simulink model "s23"  (R2019b)
settings: Solver=VariableStepAuto  StartTime=0.0  StopTime=10.0  RelTol=1e-3
values from neighbouring files (symbols this model uses):
  D = DVect(2)    [aula3.m]    (also in aula3_mica.m = Dvector(n); s23.m = 0.1)
  J = Jl + Jm    [s23.m]
  Km = 1 ,Kg = 0.1    [s23.m]
  L = 1e-3    (= 0.001)    [ex1.m]
  R = 10    [ex1.m]
undefined symbols (not defined in the file or in its folder): Kg
settings Model: Creator=Emanuel Pereira  LastModifiedBy=Emanuel Pereira

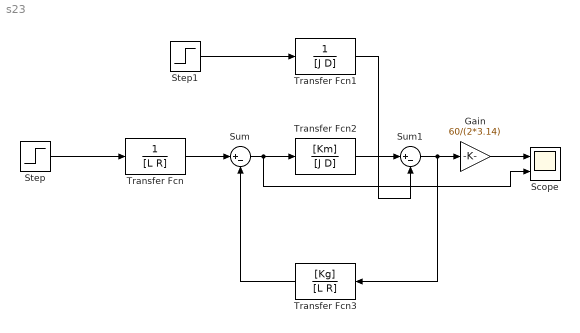
== system s23 ==
  Gain : Gain  Gain=60/(2*3.14)
  Scope : Scope  NumInputPorts=2
  Step : Step  Time=0  After=10  SampleTime=0
  Step1 : Step  Time=50  After=5  SampleTime=0
  Sum : Sum  Inputs=|+-
  Sum1 : Sum  Inputs=|+-
  Transfer Fcn : TransferFcn  Denominator=[L R]
  Transfer Fcn1 : TransferFcn  Denominator=[J D]
  Transfer Fcn2 : TransferFcn  Numerator=[Km]  Denominator=[J D]
  Transfer Fcn3 : TransferFcn  Numerator=[Kg]  Denominator=[L R]
  wires:
  Step/1 -> Transfer Fcn/1
  Transfer Fcn/1 -> Sum/1
  Sum/1 -> Scope/2, Transfer Fcn2/1
  Transfer Fcn2/1 -> Sum1/1
  Sum1/1 -> Transfer Fcn3/1, Gain/1
  Step1/1 -> Transfer Fcn1/1
  Transfer Fcn3/1 -> Sum/2
  Transfer Fcn1/1 -> Sum1/2
  Gain/1 -> Scope/1
